simulink model "windEmulatorStep3"  (R2021a)
settings: Solver=ode4  StartTime=0.0  StopTime=inf  FixedStep=0.002  RelTol=1e-3
values from neighbouring files (symbols this model uses):
  ctrlModeSpeed = logical(false)    [initStep4.m]
  ctrlModeTorque = logical(true)    [initStep4.m]
  Dm_max = 40    [initStep4.m]
  EffMechMax = 0.93    [initStep4.m]
  EffMechMin = 0.79    [initStep4.m]
  FactorEff = psi2pa*cc2m3*(1/rev2rad)    (= 0.00109733470463)    [initStep4.m]
  genMaxTorque = 0.975*acs880RatedTorque    (= 78.48165)    [initStep4.m]
  Kdamping = -500    [OptimizationResultsLoad.m]
  Kpos = 0    [OptimizationResultsLoad.m]
  nPreDrop = 2900    [initStep4.m]
  nPreDropMin = 725    [initStep4.m]
  StatusWord = bitset(StatusWord,16)    [VFD_StatusWord.m]
  T = 4    [initStep4.m]
  wheelRadius = targetWaveBotVel/targetOmega    (= 0.00477464829276)    [initStep4.m]
undefined symbols (not defined in the file or in its folder): ACS880PILimLo, ACS880PILimUp, DiscIntNeverNeededParam, Gen_REF2_Max, Gen_SpeedScaling, minPressureRef, Motor_SpeedScaling, Motor_TorqueScaling, PressureControl, ratedTorque, rpm2rps, SpeedControl, speedScalingACS800, TorqueFieldbusScale, TorqueInputControl, TorqueRefMin
libraries: fl_lib x41, nesl_utility x24, slrealtimeethercatlib x21, sh_lib x16, cstblocks x4, simulink x3, pid_lib x3, sdl_lib x1, dspstat3 x1
(part 2 of 3)

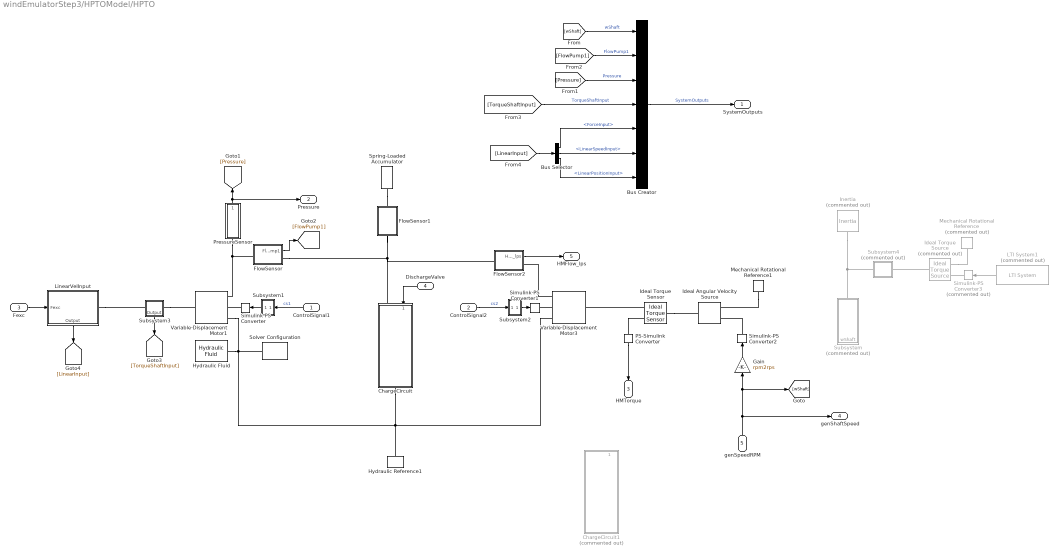
== system windEmulatorStep3/HPTOModel/HPTO ==
  ControlSignal1 : Inport
  ControlSignal2 : Inport  Port=2
  Fexc : Inport  Port=3
  DischargeValve : Inport  Port=4
  genSpeedRPM : Inport  Port=5
  Bus Creator : BusCreator  Inputs=7
  Bus Selector : BusSelector  OutputSignals=ForceInput,LinearSpeedInput,LinearPositionInput
  ChargeCircuit : Subsystem
      settings: PortSchema="{\"entries\":[{\"content\":{\"sides\":[{\"content\":{\"connectorIds\":[\"LConn1\",\"In1\"]},\"type\":\"ConnectorPlacement.EquallySpacedRectSide\",\"uuid\":\"82d1daf8-710b-4985-b266-be1c706fd037\"},{\"content\":{\"connectorIds\":[\"RConn1\"],\"side\":\"RIGHT\"},\"type\":\"ConnectorPlacement.EquallySpacedRectSide\",\"uuid\":\"cd9d67f9-1549-4eed-bef0-0a9dd1fc786d\"},{\"content\":{\"connectorIds\":[],\"side\":\"TOP\"},\"type\":\"ConnectorPlacement.EquallySpacedRectSide\",\"uuid\":\"e41a24c3-7fe9-4850-b669-e053dd15bed4\"},{\"content\":{\"connectorIds\":[],\"side\":\"BOTTOM\"},\"type\":\"ConnectorPlacement.EquallySpacedRectSide\",\"uuid\":\"127c729b-2c4a-40cb-ada2-aa7d7979a424\"}]},\"type\":\"ConnectorPlacement.EquallySpacedConnector\",\"uuid\":\"9c677d2b-4aa8-4aee-a320-3219a43d5bc8\"}],\"packageUris\":[\"http://schema.mathworks.com/mf0/Connector/R2020b\"],\"version\":\"1.0\"}"
  ChargeCircuit1 : Subsystem  Commented=on
      settings: PortSchema="{\"entries\":[{\"content\":{\"sides\":[{\"content\":{\"connectorIds\":[\"LConn1\",\"In1\"]},\"type\":\"ConnectorPlacement.EquallySpacedRectSide\",\"uuid\":\"82d1daf8-710b-4985-b266-be1c706fd037\"},{\"content\":{\"connectorIds\":[\"RConn1\"],\"side\":\"RIGHT\"},\"type\":\"ConnectorPlacement.EquallySpacedRectSide\",\"uuid\":\"cd9d67f9-1549-4eed-bef0-0a9dd1fc786d\"},{\"content\":{\"connectorIds\":[],\"side\":\"TOP\"},\"type\":\"ConnectorPlacement.EquallySpacedRectSide\",\"uuid\":\"e41a24c3-7fe9-4850-b669-e053dd15bed4\"},{\"content\":{\"connectorIds\":[\"RConn2\"],\"side\":\"BOTTOM\"},\"type\":\"ConnectorPlacement.EquallySpacedRectSide\",\"uuid\":\"127c729b-2c4a-40cb-ada2-aa7d7979a424\"}]},\"type\":\"ConnectorPlacement.EquallySpacedConnector\",\"uuid\":\"9c677d2b-4aa8-4aee-a320-3219a43d5bc8\"}],\"packageUris\":[\"http://schema.mathworks.com/mf0/Connector/R2020b\"],\"version\":\"1.0\"}"
  FlowSensor : Subsystem
  FlowSensor1 : Subsystem
  FlowSensor2 : Subsystem
  Gain : Gain  Gain=rpm2rps
  Hydraulic Fluid : sh_lib/Hydraulic Utilities/Hydraulic Fluid  DataSource=1  SelFluid=1  SysTemp=60  TrapAir=0.005  ViscDerFactor=1  range_error=1
  Hydraulic Reference1 : fl_lib/Hydraulic/Hydraulic Elements/Hydraulic Reference
  Ideal Angular Velocity Source : fl_lib/Mechanical/Mechanical Sources/Ideal Angular Velocity Source
  Ideal Torque Sensor : fl_lib/Mechanical/Mechanical Sensors/Ideal Torque Sensor
  Ideal Torque Source : fl_lib/Mechanical/Mechanical Sources/Ideal Torque Source  Commented=on
  Inertia : fl_lib/Mechanical/Rotational Elements/Inertia  Commented=on  inertia=1 kg*m^2  num_ports=foundation.enum.numPorts2.one  w_specify=off  w_priority=High  w=0 rpm  w_nominal_specify=off  w_nominal_unit=rad/s  w_nominal_value=1  t_specify=off  t_priority=None  t=0 N*m  t_nominal_specify=off  t_nominal_unit=N*m  t_nominal_value=1
  LTI System1 : cstblocks/LTI System  Commented=on  sys=tf(100*2*pi,[1 200*pi])  IC=[]
  LinearVelInput : Subsystem
      settings: PortSchema="{\"entries\":[{\"content\":{\"sides\":[{\"content\":{\"connectorIds\":[\"LConn1\"]},\"type\":\"ConnectorPlacement.EquallySpacedRectSide\",\"uuid\":\"4859a0f7-9f9b-474b-bb49-bd256c408622\"},{\"content\":{\"connectorIds\":[\"In1\"],\"side\":\"RIGHT\"},\"type\":\"ConnectorPlacement.EquallySpacedRectSide\",\"uuid\":\"5e25e59b-8f8b-4773-b6d9-951d4129523a\"},{\"content\":{\"connectorIds\":[],\"side\":\"TOP\"},\"type\":\"ConnectorPlacement.EquallySpacedRectSide\",\"uuid\":\"bae24e3d-e286-4bf4-a21b-122b1e5bc09f\"},{\"content\":{\"connectorIds\":[\"Out1\"],\"side\":\"BOTTOM\"},\"type\":\"ConnectorPlacement.EquallySpacedRectSide\",\"uuid\":\"0ce66b8b-3f3a-4f1a-9606-df56b31d9b3c\"}]},\"type\":\"ConnectorPlacement.EquallySpacedConnector\",\"uuid\":\"f87c39b6-c8d4-4afb-9096-6dab01ec5afa\"}],\"packageUris\":[\"http://schema.mathworks.com/mf0/Connector/R2020b\"],\"version\":\"1.0\"}"
  Mechanical Rotational Reference : fl_lib/Mechanical/Rotational Elements/Mechanical Rotational Reference  Commented=on
  Mechanical Rotational Reference1 : fl_lib/Mechanical/Rotational Elements/Mechanical Rotational Reference
  PS-Simulink Converter : nesl_utility/PS-Simulink Converter  PhysicalDomain=network_engine_domain  SubClassName=ps_output  LeftPortType=input  RightPortType=output  PseudoPeriodic=off  Frequencies=[]  Unit=inherit  AffineConversion=off
      settings: SourceProductBaseCode=PW,SS
  PressureSensor : Subsystem
  Simulink-PS Converter : nesl_utility/Simulink-PS Converter  PhysicalDomain=network_engine_domain  SubClassName=ps_input  LeftPortType=input  RightPortType=output  PseudoPeriodic=off  Frequencies=[]  NoiseDistribution=none  NoiseParameters=[]  Unit=1  AffineConversion=off  FilteringAndDerivatives=provide  SimscapeFilterOrder=1  InputFilterTimeConstant=0.001  UdotUserProvided=0
      settings: SourceProductBaseCode=PW,SS
  Simulink-PS Converter1 : nesl_utility/Simulink-PS Converter  PhysicalDomain=network_engine_domain  SubClassName=ps_input  LeftPortType=input  RightPortType=output  PseudoPeriodic=off  Frequencies=[]  NoiseDistribution=none  NoiseParameters=[]  Unit=1  AffineConversion=off  FilteringAndDerivatives=provide  SimscapeFilterOrder=1  InputFilterTimeConstant=0.001  UdotUserProvided=0
      settings: SourceProductBaseCode=PW,SS
  Simulink-PS Converter2 : nesl_utility/Simulink-PS Converter  PhysicalDomain=network_engine_domain  SubClassName=ps_input  LeftPortType=input  RightPortType=output  PseudoPeriodic=off  Frequencies=[]  NoiseDistribution=none  NoiseParameters=[]  Unit=1  AffineConversion=off  FilteringAndDerivatives=provide  SimscapeFilterOrder=1  InputFilterTimeConstant=0.001  UdotUserProvided=0
      settings: SourceProductBaseCode=PW,SS
  Simulink-PS Converter3 : nesl_utility/Simulink-PS Converter  Commented=on  PhysicalDomain=network_engine_domain  SubClassName=ps_input  LeftPortType=input  RightPortType=output  PseudoPeriodic=off  Frequencies=[]  NoiseDistribution=none  NoiseParameters=[]  Unit=1  AffineConversion=off  FilteringAndDerivatives=provide  SimscapeFilterOrder=1  InputFilterTimeConstant=0.001  UdotUserProvided=0
      settings: SourceProductBaseCode=PW,SS
  Solver Configuration : nesl_utility/Solver Configuration  PhysicalDomain=network_engine_domain  SubClassName=solver  LeftPortType=input  RightPortType=generic  Tones=[]  Harmonics=[]  SimulateNoise=off  Profile=off  UseLocalSampling=off  EnableSwitchedLinearOptims=on  FrequencyDomain=off  UseCCode=off  RelTol=0.001  AbsTol=1e-06  MinStep=1e-09  ToWorkspace=off  RevertToSquareIcSolve=off  NumHomotopyIterations=100  PhasorMode=off  PhasorModeNumHarmonics=1  DoDC=off  ResidualTolerance=1e-09  UseLocalSolver=on  LocalSolverChoice=NE_BACKWARD_EULER_ADVANCER  LocalSolverSampleTime=SampleTime  DoFixedCost=on  MaxNonlinIter=3  MaxModeIter=2  ComputeImpulses=off  ImpulseIterations=2  LinearAlgebra=auto  EquationFormulation=NE_TIME_EF  DelaysMemoryBudget=1024  AutomaticFiltering=on  FilteringTimeConstant=0.001  PartitionStorageMethod=AS_NEEDED  PartitionMemoryBudget=1024  PartitionMethod=ROBUST
      settings: SourceProductBaseCode=PW,SS
  Spring-Loaded Accumulator : sh_lib/Accumulators/Spring-Loaded Accumulator  capacity=AccVol m^3  pr_preload=Acc_PC psi  pr_max=Acc_MaxP psi  stiff_coeff=1e10 Pa/m^3  penetr_coeff=1e10 Pa*s/m^6  flow_rate_specify=off  flow_rate_priority=None  flow_rate=5e-3 m^3/s  flow_rate_nominal_specify=off  flow_rate_nominal_unit=m^3/s  flow_rate_nominal_value=1  fluid_volume_specify=on  fluid_volume_priority=None  fluid_volume=5e-6 m^3  fluid_volume_nominal_specify=off  fluid_volume_nominal_unit=m^3  fluid_volume_nominal_value=1  fluid_pressure_specify=off  fluid_pressure_priority=None  fluid_pressure=1.01325e5 Pa  fluid_pressure_nominal_specify=off  fluid_pressure_nominal_unit=Pa  fluid_pressure_nominal_value=1
      settings: SourceProductBaseCode=SH  InternalSimscapePortConfiguration="{\"Bottom\":[],\"Left\":[],\"Right\":[{\"id\":\"A\",\"label\":\"A\",\"type\":\"foundation.hydraulic.hydraulic\"}],\"Top\":[]}"
  Subsystem : Subsystem  Commented=on
  Subsystem1 : Subsystem
  Subsystem2 : Subsystem
  Subsystem3 : Subsystem
      settings: PortSchema="{\"entries\":[{\"content\":{\"sides\":[{\"content\":{\"connectorIds\":[\"LConn1\"]},\"type\":\"ConnectorPlacement.EquallySpacedRectSide\",\"uuid\":\"7d5827d5-19d2-449a-bfe5-3899d5f2f234\"},{\"content\":{\"connectorIds\":[\"RConn1\"],\"side\":\"RIGHT\"},\"type\":\"ConnectorPlacement.EquallySpacedRectSide\",\"uuid\":\"27ad7fb5-d235-43aa-a783-09c3ddbf3629\"},{\"content\":{\"connectorIds\":[],\"side\":\"TOP\"},\"type\":\"ConnectorPlacement.EquallySpacedRectSide\",\"uuid\":\"41db419c-7193-454e-a54e-cfb74ab94a84\"},{\"content\":{\"connectorIds\":[\"Out1\"],\"side\":\"BOTTOM\"},\"type\":\"ConnectorPlacement.EquallySpacedRectSide\",\"uuid\":\"63d69fbc-18e5-4f7b-99db-9fcc8740eddf\"}]},\"type\":\"ConnectorPlacement.EquallySpacedConnector\",\"uuid\":\"1d29a5fa-8394-444f-93a2-8698ce035363\"}],\"packageUris\":[\"http://schema.mathworks.com/mf0/Connector/R2020b\"],\"version\":\"1.0\"}"
  Subsystem4 : Subsystem  Commented=on
  Variable-Displacement Motor1 : sh_lib/Pumps and Motors/Variable-Displacement Motor  mdl_type=2  stroke_max=0.005 m  D_max=Dm_max cm^3/rev  cntrl_mem_tab=[-.0075, 0, .0075] m  displ_tab=[-Dm_max, 0, Dm_max] cm^3/rev  interp_method=1  extrap_method=1  loss_spec=1  w_nominal=nShaftSpeed rpm  pr_nominal=nPreDrop psi  visc_nominal=18 cSt  dens_nominal=900 kg/m^3  efficiency_vol=EffVolNom  no_load_torque=nTorqueNoLoad N*m  torque_pressure_coeff=(1/((200-50)*1e5))*Dm_max*FactorEff*((1-EffMechMax)*nPreDrop-(1-EffMechMin)*nPreDropMin) N*m/Pa  p_diff_eff_TLU=[100000, 1000000, 2000000] Pa  omega_eff_TLU=[25, 50, 100, 200, 300, 400] rad/s  displacement_eff_TLU=[-30, -19, 19, 30] cm^3/rev  vol_eff_TLU=repmat([.816, .908, .954, .977, .981, .984; .325, .663, .831, .916, .925, .946; .137, .568, .78, .892, .893, .91], 1, 1, 4)  mech_eff_TLU=repmat([.996, .996, .996, .996, .996, .996; .988, .989, .989, .989, .989, .99; .981, .981, .982, .982, .983, .984], 1, 1, 4)  p_diff_loss_TLU=[100000, 1000000, 2000000] Pa  omega_loss_TLU=[25, 50, 100, 200, 300, 400] rad/s  displacement_loss_TLU=[-30, -19, 19, 30] cm^3/rev  vol_loss_TLU=repmat([.0282, .0253, .0241, .0235, .0291, .0325; .2596, .1271, .1017, .0917, .1216, .1142; .7874, .1901, .141, .1211, .1797, .1978] * 1e-3, 1, 1, 4) m^3/s  mech_loss_TLU=repmat([.002, .002, .002, .002, .002, .002; .06, .055, .055, .055, .055, .05; .19, .19, .18, .18, .17, .16], 1, 1, 4) N*m  pressure_threshold=1e5 Pa  omega_threshold=10 rad/s  displacement_threshold=0.0001 cm^3/rev  octant_check=0  pressure_check=0  min_valid_pressure=0 Pa  vol_eff_min=1e-3  vol_eff_max=1  mech_eff_min=1e-3  mech_eff_max=1
      settings: SourceProductBaseCode=SH  InternalSimscapePortConfiguration="{\"Bottom\":[],\"Left\":[{\"id\":\"A\",\"label\":\"A\",\"type\":\"foundation.hydraulic.hydraulic\"},{\"id\":\"C\",\"label\":\"C\",\"type\":\"input\"},{\"id\":\"B\",\"label\":\"B\",\"type\":\"foundation.hydraulic.hydraulic\"}],\"Right\":[{\"id\":\"S\",\"label\":\"S\",\"type\":\"foundation.mechanical.rotational.rotational\"}],\"Top\":[]}"
  Variable-Displacement Motor3 : sh_lib/Pumps and Motors/Variable-Displacement Motor  mdl_type=2  stroke_max=0.005 m  D_max=Dm_max cm^3/rev  cntrl_mem_tab=[-.0075, 0, .0075] m  displ_tab=[-Dm_max, 0, Dm_max] cm^3/rev  interp_method=1  extrap_method=1  loss_spec=1  w_nominal=nShaftSpeed rpm  pr_nominal=nPreDrop psi  visc_nominal=18 cSt  dens_nominal=900 kg/m^3  efficiency_vol=EffVolNom  no_load_torque=nTorqueNoLoad N*m  torque_pressure_coeff=(1/((200-50)*1e5))*Dm_max*FactorEff*((1-EffMechMax)*nPreDrop-(1-EffMechMin)*nPreDropMin) N*m/Pa  p_diff_eff_TLU=[100000, 1000000, 2000000] Pa  omega_eff_TLU=[25, 50, 100, 200, 300, 400] rad/s  displacement_eff_TLU=[-30, -19, 19, 30] cm^3/rev  vol_eff_TLU=repmat([.816, .908, .954, .977, .981, .984; .325, .663, .831, .916, .925, .946; .137, .568, .78, .892, .893, .91], 1, 1, 4)  mech_eff_TLU=repmat([.996, .996, .996, .996, .996, .996; .988, .989, .989, .989, .989, .99; .981, .981, .982, .982, .983, .984], 1, 1, 4)  p_diff_loss_TLU=[100000, 1000000, 2000000] Pa  omega_loss_TLU=[25, 50, 100, 200, 300, 400] rad/s  displacement_loss_TLU=[-30, -19, 19, 30] cm^3/rev  vol_loss_TLU=repmat([.0282, .0253, .0241, .0235, .0291, .0325; .2596, .1271, .1017, .0917, .1216, .1142; .7874, .1901, .141, .1211, .1797, .1978] * 1e-3, 1, 1, 4) m^3/s  mech_loss_TLU=repmat([.002, .002, .002, .002, .002, .002; .06, .055, .055, .055, .055, .05; .19, .19, .18, .18, .17, .16], 1, 1, 4) N*m  pressure_threshold=1e5 Pa  omega_threshold=10 rad/s  displacement_threshold=0.00001 cm^3/rev  octant_check=0  pressure_check=0  min_valid_pressure=0 Pa  vol_eff_min=1e-3  vol_eff_max=1  mech_eff_min=1e-3  mech_eff_max=1
      settings: SourceProductBaseCode=SH  InternalSimscapePortConfiguration="{\"Bottom\":[],\"Left\":[{\"id\":\"A\",\"label\":\"A\",\"type\":\"foundation.hydraulic.hydraulic\"},{\"id\":\"C\",\"label\":\"C\",\"type\":\"input\"},{\"id\":\"B\",\"label\":\"B\",\"type\":\"foundation.hydraulic.hydraulic\"}],\"Right\":[{\"id\":\"S\",\"label\":\"S\",\"type\":\"foundation.mechanical.rotational.rotational\"}],\"Top\":[]}"
  SystemOutputs : Outport
  Pressure : Outport  Port=2
  HMTorque : Outport  Port=3
  genShaftSpeed : Outport  Port=4
  HMFlow_lps : Outport  Port=5
  wires:
  LTI System1/1 -> Simulink-PS Converter3/1
  [wShaft] -> Bus Creator/1  "wShaft"
  PressureSensor/1(Pressure) -> Pressure/1, [Pressure]
  Bus Creator/1 -> SystemOutputs/1  "SystemOutputs"
  ControlSignal1/1 -> Subsystem1/1(In1)  "cs1"
  Subsystem1/1(Out1) -> Simulink-PS Converter/1
  Subsystem2/1(Out1) -> Simulink-PS Converter1/1
  ControlSignal2/1 -> Subsystem2/1(1)  "cs2"
  FlowSensor/1(FlowPump1) -> [FlowPump1]
  [FlowPump1] -> Bus Creator/2  "FlowPump1"
  [Pressure] -> Bus Creator/3  "Pressure"
  Subsystem3/1(Output) -> [TorqueShaftInput]
  [TorqueShaftInput] -> Bus Creator/4  "TorqueShaftInput"
  LinearVelInput/1(Output) -> [LinearInput]
  [LinearInput] -> Bus Selector/1
  Bus Selector/2 -> Bus Creator/6  "<LinearSpeedInput>"
  Bus Selector/1 -> Bus Creator/5  "<ForceInput>"
  Bus Selector/3 -> Bus Creator/7  "<LinearPositionInput>"
  Fexc/1 -> LinearVelInput/1(Fexc)
  DischargeValve/1 -> ChargeCircuit/1(DischargeValve)
  Gain/1 -> Simulink-PS Converter2/1
  genSpeedRPM/1 -> [wShaft], Gain/1, genShaftSpeed/1
  PS-Simulink Converter/1 -> HMTorque/1
  FlowSensor2/1(HMFlow_lps) -> HMFlow_lps/1
  connections:
  Subsystem/LConn1 -- Subsystem4/RConn1 -- Inertia/LConn1
  FlowSensor1/LConn1 -- ChargeCircuit/LConn1 -- FlowSensor2/LConn1 -- FlowSensor/RConn1
  PressureSensor/LConn1 -- Variable-Displacement Motor1/LConn1 -- FlowSensor/LConn1
  Ideal Torque Source/RConn2 -- Mechanical Rotational Reference/LConn1
  Simulink-PS Converter3/RConn1 -- Ideal Torque Source/RConn1
  Variable-Displacement Motor3/LConn2 -- Simulink-PS Converter1/RConn1
  Simulink-PS Converter/RConn1 -- Variable-Displacement Motor1/LConn2
  Spring-Loaded Accumulator/RConn1 -- FlowSensor1/RConn1
  Variable-Displacement Motor3/LConn1 -- FlowSensor2/RConn1
  Subsystem3/RConn1 -- Variable-Displacement Motor1/RConn1
  LinearVelInput/LConn1 -- Subsystem3/LConn1
  Ideal Torque Source/LConn1 -- Subsystem4/LConn1
  Variable-Displacement Motor1/LConn3 -- Hydraulic Reference1/LConn1 -- ChargeCircuit/RConn1 -- Variable-Displacement Motor3/LConn3 -- Solver Configuration/RConn1 -- Hydraulic Fluid/RConn1
  Simulink-PS Converter2/RConn1 -- Ideal Angular Velocity Source/RConn1
  Mechanical Rotational Reference1/LConn1 -- Ideal Angular Velocity Source/RConn2
  Ideal Torque Sensor/LConn1 -- Ideal Angular Velocity Source/LConn1
  Ideal Torque Sensor/RConn1 -- Variable-Displacement Motor3/RConn1
  PS-Simulink Converter/LConn1 -- Ideal Torque Sensor/RConn2

== system windEmulatorStep3/HPTOModel/ControlAlgorithm/ForceToTorque ==
  ActualSignals : Inport
  Bus Selector : BusSelector  OutputSignals=LinearSpeedInput,LinearPositionInput
  Constant2 : Constant  Value=wheelRadius
  DesiredForce : Subsystem
  Gain : Gain  Gain=-1
  Product2 : Product
  TorqueD : Outport
  wires:
  ActualSignals/1 -> Bus Selector/1
  Product2/1 -> Gain/1
  Constant2/1 -> Product2/2
  Bus Selector/1 -> DesiredForce/1(<LinearSpeedInput>)  "<LinearSpeedInput>"
  Bus Selector/2 -> DesiredForce/2(<LinearPositionInput>)  "<LinearPositionInput>"
  DesiredForce/1(ForceD) -> Product2/1
  Gain/1 -> TorqueD/1

== system windEmulatorStep3/HPTOModel/ControlAlgorithm/PressureAbovePmin ==
  ActualSignals : Inport
  RefValues : Inport  Port=2
  SpeedControllerReset : Inport  Port=3
  Bus Selector : BusSelector  OutputSignals=TorqueShaftInput,Pressure,wShaft
  Bus Selector1 : BusSelector  OutputSignals=TorqueInputRef,PressureRef,SheftSpeedRef
  PressureControl1 : Subsystem
  SpeedControl1 : Subsystem
  Terminator1 : Terminator
  TorqueControl1 : Subsystem
  ControlSignal1 : Outport
  ControlSignal2 : Outport  Port=2
  ControlTorqueLoad : Outport  Port=3
  wires:
  ActualSignals/1 -> Bus Selector/1
  TorqueControl1/1(ControlSignal1) -> ControlSignal1/1
  Bus Selector/3 -> SpeedControl1/1(ShaftSpeedMotor)  "<wShaft>"
  RefValues/1 -> Bus Selector1/1
  Bus Selector1/1 -> TorqueControl1/1(TorqueRef)  "<TorqueInputRef>"
  Bus Selector1/3 -> SpeedControl1/2(ShaftSpeedRef)  "<SheftSpeedRef>"
  PressureControl1/1(ControlSignal2) -> ControlSignal2/1
  Bus Selector/2 -> PressureControl1/1(ActualPressure)  "<Pressure>"
  Bus Selector/1 -> Terminator1/1  "<TorqueShaftInput>"
  Bus Selector1/2 -> PressureControl1/2(PressureRef)  "<PressureRef>"
  SpeedControl1/1(ContolTorque) -> ControlTorqueLoad/1
  SpeedControllerReset/1 -> SpeedControl1/3(SpeedControllerReset)

== system windEmulatorStep3/HPTOModel/ControlAlgorithm/PressureBelowPmin ==
  ActualSignals : Inport
  RefValues : Inport  Port=2
  SpeedControllerReset : Inport  Port=3
  Bus Selector : BusSelector  OutputSignals=TorqueShaftInput,Pressure,wShaft
  Bus Selector1 : BusSelector  OutputSignals=TorqueInputRef,PressureRef,SheftSpeedRef
  PressureControl1 : Subsystem
  SpeedControl1 : Subsystem
  TorqueControl1 : Subsystem
  ControlSignal1 : Outport
  ControlSignal2 : Outport  Port=2
  ControlTorqueLoad : Outport  Port=3
  wires:
  ActualSignals/1 -> Bus Selector/1
  Bus Selector/1 -> TorqueControl1/1(ActualTorqueInput)  "<TorqueShaftInput>"
  TorqueControl1/1(ControlSignal1) -> ControlSignal1/1
  PressureControl1/1(ControlSignal2) -> ControlSignal2/1
  Bus Selector/2 -> TorqueControl1/3(Pressure), PressureControl1/1(ActualPressure)  "<Pressure>"
  Bus Selector/3 -> SpeedControl1/1(ShaftSpeedMotor)  "<wShaft>"
  SpeedControl1/1(ContolTorque) -> ControlTorqueLoad/1
  RefValues/1 -> Bus Selector1/1
  Bus Selector1/1 -> TorqueControl1/2(TorqueRef)  "<TorqueInputRef>"
  Bus Selector1/2 -> PressureControl1/2(PressureRef)  "<PressureRef>"
  Bus Selector1/3 -> SpeedControl1/2(ShaftSpeedRef)  "<SheftSpeedRef>"
  SpeedControllerReset/1 -> SpeedControl1/3(SpeedControllerReset)

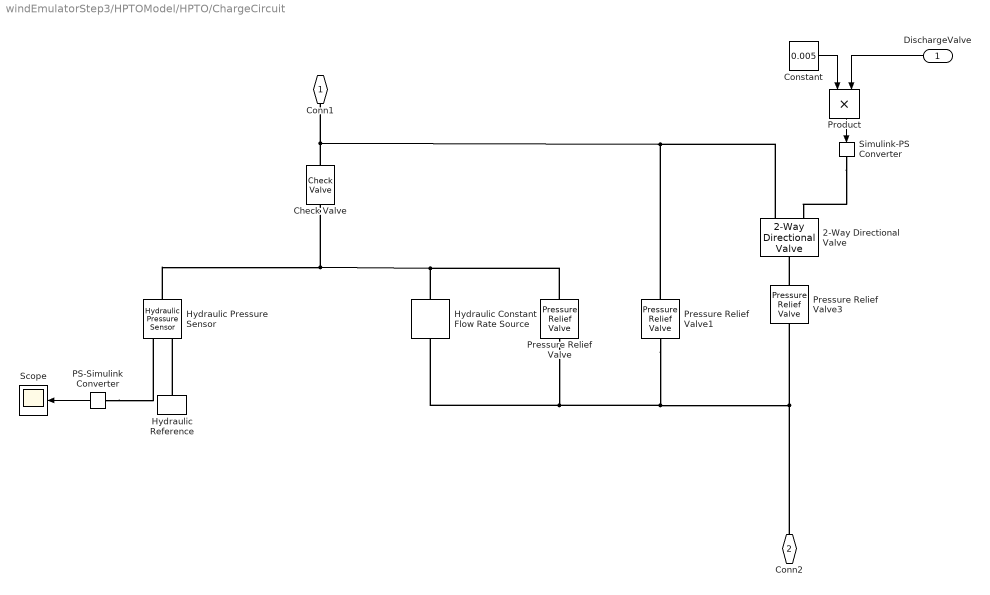
== system windEmulatorStep3/HPTOModel/HPTO/ChargeCircuit ==
  DischargeValve : Inport
  2-Way Directional Valve : sh_lib/Valves/Directional Valves/2-Way Directional Valve  mdl_type=1  area_max=0.5e-4 m^2  opening_max=0.005 m  opening_tab=[-.002, 0, .002, .005, .015] m  area_tab=[1e-09, 2.0352e-07, 4.0736e-05, .00011438, .00034356] m^2  pressure_tab=[-10000000, -5000000, -2000000, 2000000, 5000000, 10000000] Pa  flow_rate_tab=[-1e-07, -7.0711e-08, -4.4721e-08, 4.4721e-08, 7.0711e-08, 1e-07; -2.0352e-05, -1.4391e-05, -9.1017e-06, 9.1017e-06, 1.4391e-05, 2.0352e-05; -.0040736, -.0028805, -.0018218, .0018218, .0028805, .0040736; -.011438, -.0080879, -.0051152, .0051152, .0080879, .011438; -.034356, -.024293, -.015364, .015364, .024293, .034356] m^3/s  interp_method=1  extrap_method=1  C_d=0.7  x_0=0 m  A_leak=1e-12 m^2  lam_spec=1  B_lam=0.999  Re_cr=12
      settings: SourceProductBaseCode=SH  InternalSimscapePortConfiguration="{\"Bottom\":[],\"Left\":[{\"id\":\"S\",\"label\":\"S\",\"type\":\"input\"},{\"id\":\"A\",\"label\":\"A\",\"type\":\"foundation.hydraulic.hydraulic\"}],\"Right\":[{\"id\":\"B\",\"label\":\"B\",\"type\":\"foundation.hydraulic.hydraulic\"}],\"Top\":[]}"
  Check Valve : sh_lib/Valves/Directional Valves/Check Valve  area_max=1e-4 m^2  pres_crack=0.3e5 Pa  pres_max=1.2e5 Pa  C_d=0.7  A_leak=1e-12 m^2  lam_spec=1  B_lam=0.999  Re_cr=12  dynamic=0  tau=0.1 s  area_init=1e-12 m^2
      settings: SourceProductBaseCode=SH  InternalSimscapePortConfiguration="{\"Bottom\":[],\"Left\":[{\"id\":\"A\",\"label\":\"A\",\"type\":\"foundation.hydraulic.hydraulic\"}],\"Right\":[{\"id\":\"B\",\"label\":\"B\",\"type\":\"foundation.hydraulic.hydraulic\"}],\"Top\":[]}"
  Constant : Constant  Value=0.005
  Hydraulic Constant Flow Rate Source : fl_lib/Hydraulic/Hydraulic Sources/Hydraulic Constant Flow Rate Source  commanded_flow_rate=5 lpm
      settings: SourceProductBaseCode=SS  InternalSimscapePortConfiguration="{\"Bottom\":[],\"Left\":[{\"id\":\"P\",\"label\":\"P\",\"type\":\"foundation.hydraulic.hydraulic\"}],\"Right\":[{\"id\":\"T\",\"label\":\"T\",\"type\":\"foundation.hydraulic.hydraulic\"}],\"Top\":[]}"
  Hydraulic Pressure Sensor : fl_lib/Hydraulic/Hydraulic Sensors/Hydraulic Pressure Sensor
  Hydraulic Reference : fl_lib/Hydraulic/Hydraulic Elements/Hydraulic Reference
  PS-Simulink Converter : nesl_utility/PS-Simulink Converter  PhysicalDomain=network_engine_domain  SubClassName=ps_output  LeftPortType=input  RightPortType=output  PseudoPeriodic=off  Frequencies=[]  Unit=inherit  AffineConversion=off
      settings: SourceProductBaseCode=PW,SS
  Pressure Relief Valve : sh_lib/Valves/Pressure Control Valves/Pressure Relief Valve  valve_area_spec=1  p_diff_TLU=[30.15e5 : 15e3 : 31.35e5] Pa  area_TLU=[1 : 1 : 9] .* 1e-5 m^2  area_max=1e-4 m^2  pres_set=10 psi  reg_range=5 psi  C_d=0.7  A_leak=1e-12 m^2  lam_spec=1  B_lam=0.999  Re_cr=12  dynamic=0  tau=0.1 s  area_init=1e-12 m^2
      settings: SourceProductBaseCode=SH  InternalSimscapePortConfiguration="{\"Bottom\":[],\"Left\":[{\"id\":\"A\",\"label\":\"A\",\"type\":\"foundation.hydraulic.hydraulic\"}],\"Right\":[{\"id\":\"B\",\"label\":\"B\",\"type\":\"foundation.hydraulic.hydraulic\"}],\"Top\":[]}"
  Pressure Relief Valve1 : sh_lib/Valves/Pressure Control Valves/Pressure Relief Valve  valve_area_spec=1  p_diff_TLU=[30.15e5 : 15e3 : 31.35e5] Pa  area_TLU=[1 : 1 : 9] .* 1e-5 m^2  area_max=1e-4 m^2  pres_set=PressureValveMax psi  reg_range=ValvePreRange psi  C_d=0.7  A_leak=1e-12 m^2  lam_spec=1  B_lam=0.999  Re_cr=12  dynamic=0  tau=0.1 s  area_init=1e-12 m^2
      settings: SourceProductBaseCode=SH  InternalSimscapePortConfiguration="{\"Bottom\":[],\"Left\":[{\"id\":\"A\",\"label\":\"A\",\"type\":\"foundation.hydraulic.hydraulic\"}],\"Right\":[{\"id\":\"B\",\"label\":\"B\",\"type\":\"foundation.hydraulic.hydraulic\"}],\"Top\":[]}"
  Pressure Relief Valve3 : sh_lib/Valves/Pressure Control Valves/Pressure Relief Valve  valve_area_spec=1  p_diff_TLU=[30.15e5 : 15e3 : 31.35e5] Pa  area_TLU=[1 : 1 : 9] .* 1e-5 m^2  area_max=1e-4 m^2  pres_set=50 psi  reg_range=5 psi  C_d=0.7  A_leak=1e-12 m^2  lam_spec=1  B_lam=0.999  Re_cr=12  dynamic=0  tau=0.1 s  area_init=1e-12 m^2
      settings: SourceProductBaseCode=SH  InternalSimscapePortConfiguration="{\"Bottom\":[],\"Left\":[{\"id\":\"A\",\"label\":\"A\",\"type\":\"foundation.hydraulic.hydraulic\"}],\"Right\":[{\"id\":\"B\",\"label\":\"B\",\"type\":\"foundation.hydraulic.hydraulic\"}],\"Top\":[]}"
  Product : Product
  Scope : Scope
  Simulink-PS Converter : nesl_utility/Simulink-PS Converter  PhysicalDomain=network_engine_domain  SubClassName=ps_input  LeftPortType=input  RightPortType=output  PseudoPeriodic=off  Frequencies=[]  NoiseDistribution=none  NoiseParameters=[]  Unit=1  AffineConversion=off  FilteringAndDerivatives=provide  SimscapeFilterOrder=1  InputFilterTimeConstant=0.001  UdotUserProvided=0
      settings: SourceProductBaseCode=PW,SS
  Conn1 : PMIOPort  Side=Left
  Conn2 : PMIOPort  Port=2  Side=Right
  wires:
  PS-Simulink Converter/1 -> Scope/1
  Product/1 -> Simulink-PS Converter/1
  Constant/1 -> Product/1
  DischargeValve/1 -> Product/2
  connections:
  Hydraulic Pressure Sensor/LConn1 -- Pressure Relief Valve/LConn1 -- Hydraulic Constant Flow Rate Source/LConn1 -- Check Valve/LConn1
  Hydraulic Constant Flow Rate Source/RConn1 -- Pressure Relief Valve1/RConn1 -- Conn2/RConn1 -- Pressure Relief Valve3/RConn1 -- Pressure Relief Valve/RConn1
  Check Valve/RConn1 -- 2-Way Directional Valve/LConn2 -- Pressure Relief Valve1/LConn1 -- Conn1/RConn1
  Hydraulic Reference/LConn1 -- Hydraulic Pressure Sensor/RConn1
  PS-Simulink Converter/LConn1 -- Hydraulic Pressure Sensor/RConn2
  Simulink-PS Converter/RConn1 -- 2-Way Directional Valve/LConn1
  Pressure Relief Valve3/LConn1 -- 2-Way Directional Valve/RConn1

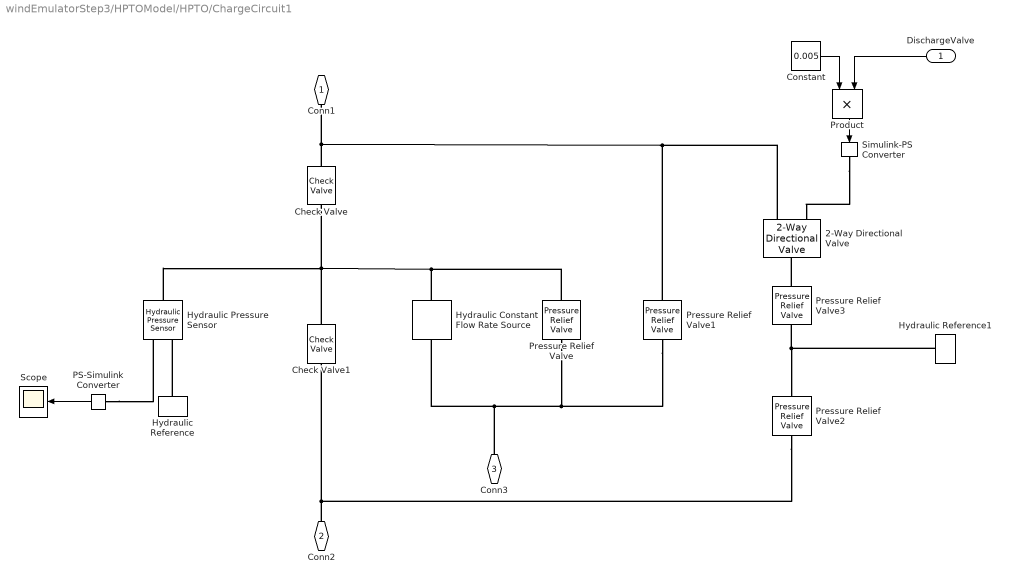
== system windEmulatorStep3/HPTOModel/HPTO/ChargeCircuit1 ==
  DischargeValve : Inport
  2-Way Directional Valve : sh_lib/Valves/Directional Valves/2-Way Directional Valve  mdl_type=1  area_max=0.5e-4 m^2  opening_max=0.005 m  opening_tab=[-.002, 0, .002, .005, .015] m  area_tab=[1e-09, 2.0352e-07, 4.0736e-05, .00011438, .00034356] m^2  pressure_tab=[-10000000, -5000000, -2000000, 2000000, 5000000, 10000000] Pa  flow_rate_tab=[-1e-07, -7.0711e-08, -4.4721e-08, 4.4721e-08, 7.0711e-08, 1e-07; -2.0352e-05, -1.4391e-05, -9.1017e-06, 9.1017e-06, 1.4391e-05, 2.0352e-05; -.0040736, -.0028805, -.0018218, .0018218, .0028805, .0040736; -.011438, -.0080879, -.0051152, .0051152, .0080879, .011438; -.034356, -.024293, -.015364, .015364, .024293, .034356] m^3/s  interp_method=1  extrap_method=1  C_d=0.7  x_0=0 m  A_leak=1e-12 m^2  lam_spec=1  B_lam=0.999  Re_cr=12
      settings: SourceProductBaseCode=SH  InternalSimscapePortConfiguration="{\"Bottom\":[],\"Left\":[{\"id\":\"S\",\"label\":\"S\",\"type\":\"input\"},{\"id\":\"A\",\"label\":\"A\",\"type\":\"foundation.hydraulic.hydraulic\"}],\"Right\":[{\"id\":\"B\",\"label\":\"B\",\"type\":\"foundation.hydraulic.hydraulic\"}],\"Top\":[]}"
  Check Valve : sh_lib/Valves/Directional Valves/Check Valve  area_max=1e-4 m^2  pres_crack=0.3e5 Pa  pres_max=1.2e5 Pa  C_d=0.7  A_leak=1e-12 m^2  lam_spec=1  B_lam=0.999  Re_cr=12  dynamic=0  tau=0.1 s  area_init=1e-12 m^2
      settings: SourceProductBaseCode=SH  InternalSimscapePortConfiguration="{\"Bottom\":[],\"Left\":[{\"id\":\"A\",\"label\":\"A\",\"type\":\"foundation.hydraulic.hydraulic\"}],\"Right\":[{\"id\":\"B\",\"label\":\"B\",\"type\":\"foundation.hydraulic.hydraulic\"}],\"Top\":[]}"
  Check Valve1 : sh_lib/Valves/Directional Valves/Check Valve  area_max=1e-4 m^2  pres_crack=0.3e5 Pa  pres_max=1.2e5 Pa  C_d=0.7  A_leak=1e-12 m^2  lam_spec=1  B_lam=0.999  Re_cr=12  dynamic=0  tau=0.1 s  area_init=1e-12 m^2
      settings: SourceProductBaseCode=SH  InternalSimscapePortConfiguration="{\"Bottom\":[],\"Left\":[{\"id\":\"A\",\"label\":\"A\",\"type\":\"foundation.hydraulic.hydraulic\"}],\"Right\":[{\"id\":\"B\",\"label\":\"B\",\"type\":\"foundation.hydraulic.hydraulic\"}],\"Top\":[]}"
  Constant : Constant  Value=0.005
  Hydraulic Constant Flow Rate Source : fl_lib/Hydraulic/Hydraulic Sources/Hydraulic Constant Flow Rate Source  commanded_flow_rate=35 lpm
      settings: SourceProductBaseCode=SS  InternalSimscapePortConfiguration="{\"Bottom\":[],\"Left\":[{\"id\":\"P\",\"label\":\"P\",\"type\":\"foundation.hydraulic.hydraulic\"}],\"Right\":[{\"id\":\"T\",\"label\":\"T\",\"type\":\"foundation.hydraulic.hydraulic\"}],\"Top\":[]}"
  Hydraulic Pressure Sensor : fl_lib/Hydraulic/Hydraulic Sensors/Hydraulic Pressure Sensor
  Hydraulic Reference : fl_lib/Hydraulic/Hydraulic Elements/Hydraulic Reference
  Hydraulic Reference1 : fl_lib/Hydraulic/Hydraulic Elements/Hydraulic Reference
  PS-Simulink Converter : nesl_utility/PS-Simulink Converter  PhysicalDomain=network_engine_domain  SubClassName=ps_output  LeftPortType=input  RightPortType=output  PseudoPeriodic=off  Frequencies=[]  Unit=inherit  AffineConversion=off
      settings: SourceProductBaseCode=PW,SS
  Pressure Relief Valve : sh_lib/Valves/Pressure Control Valves/Pressure Relief Valve  valve_area_spec=1  p_diff_TLU=[30.15e5 : 15e3 : 31.35e5] Pa  area_TLU=[1 : 1 : 9] .* 1e-5 m^2  area_max=1e-4 m^2  pres_set=50 psi  reg_range=5 psi  C_d=0.7  A_leak=1e-12 m^2  lam_spec=1  B_lam=0.999  Re_cr=12  dynamic=0  tau=0.1 s  area_init=1e-12 m^2
      settings: SourceProductBaseCode=SH  InternalSimscapePortConfiguration="{\"Bottom\":[],\"Left\":[{\"id\":\"A\",\"label\":\"A\",\"type\":\"foundation.hydraulic.hydraulic\"}],\"Right\":[{\"id\":\"B\",\"label\":\"B\",\"type\":\"foundation.hydraulic.hydraulic\"}],\"Top\":[]}"
  Pressure Relief Valve1 : sh_lib/Valves/Pressure Control Valves/Pressure Relief Valve  valve_area_spec=1  p_diff_TLU=[30.15e5 : 15e3 : 31.35e5] Pa  area_TLU=[1 : 1 : 9] .* 1e-5 m^2  area_max=1e-4 m^2  pres_set=PressureValveMax psi  reg_range=ValvePreRange psi  C_d=0.7  A_leak=1e-12 m^2  lam_spec=1  B_lam=0.999  Re_cr=12  dynamic=0  tau=0.1 s  area_init=1e-12 m^2
      settings: SourceProductBaseCode=SH  InternalSimscapePortConfiguration="{\"Bottom\":[],\"Left\":[{\"id\":\"A\",\"label\":\"A\",\"type\":\"foundation.hydraulic.hydraulic\"}],\"Right\":[{\"id\":\"B\",\"label\":\"B\",\"type\":\"foundation.hydraulic.hydraulic\"}],\"Top\":[]}"
  Pressure Relief Valve2 : sh_lib/Valves/Pressure Control Valves/Pressure Relief Valve  valve_area_spec=1  p_diff_TLU=[30.15e5 : 15e3 : 31.35e5] Pa  area_TLU=[1 : 1 : 9] .* 1e-5 m^2  area_max=1e-4 m^2  pres_set=PressureValveMax psi  reg_range=ValvePreRange psi  C_d=0.7  A_leak=1e-12 m^2  lam_spec=1  B_lam=0.999  Re_cr=12  dynamic=0  tau=0.1 s  area_init=1e-12 m^2
      settings: SourceProductBaseCode=SH  InternalSimscapePortConfiguration="{\"Bottom\":[],\"Left\":[{\"id\":\"A\",\"label\":\"A\",\"type\":\"foundation.hydraulic.hydraulic\"}],\"Right\":[{\"id\":\"B\",\"label\":\"B\",\"type\":\"foundation.hydraulic.hydraulic\"}],\"Top\":[]}"
  Pressure Relief Valve3 : sh_lib/Valves/Pressure Control Valves/Pressure Relief Valve  valve_area_spec=1  p_diff_TLU=[30.15e5 : 15e3 : 31.35e5] Pa  area_TLU=[1 : 1 : 9] .* 1e-5 m^2  area_max=1e-4 m^2  pres_set=50 psi  reg_range=5 psi  C_d=0.7  A_leak=1e-12 m^2  lam_spec=1  B_lam=0.999  Re_cr=12  dynamic=0  tau=0.1 s  area_init=1e-12 m^2
      settings: SourceProductBaseCode=SH  InternalSimscapePortConfiguration="{\"Bottom\":[],\"Left\":[{\"id\":\"A\",\"label\":\"A\",\"type\":\"foundation.hydraulic.hydraulic\"}],\"Right\":[{\"id\":\"B\",\"label\":\"B\",\"type\":\"foundation.hydraulic.hydraulic\"}],\"Top\":[]}"
  Product : Product
  Scope : Scope
  Simulink-PS Converter : nesl_utility/Simulink-PS Converter  PhysicalDomain=network_engine_domain  SubClassName=ps_input  LeftPortType=input  RightPortType=output  PseudoPeriodic=off  Frequencies=[]  NoiseDistribution=none  NoiseParameters=[]  Unit=1  AffineConversion=off  FilteringAndDerivatives=provide  SimscapeFilterOrder=1  InputFilterTimeConstant=0.001  UdotUserProvided=0
      settings: SourceProductBaseCode=PW,SS
  Conn1 : PMIOPort  Side=Left
  Conn2 : PMIOPort  Port=2  Side=Right
  Conn3 : PMIOPort  Port=3  Side=Right
  wires:
  PS-Simulink Converter/1 -> Scope/1
  Product/1 -> Simulink-PS Converter/1
  Constant/1 -> Product/1
  DischargeValve/1 -> Product/2
  connections:
  Check Valve1/LConn1 -- Hydraulic Pressure Sensor/LConn1 -- Pressure Relief Valve/LConn1 -- Hydraulic Constant Flow Rate Source/LConn1 -- Check Valve/LConn1
  Conn2/RConn1 -- Pressure Relief Valve2/LConn1 -- Check Valve1/RConn1
  Check Valve/RConn1 -- 2-Way Directional Valve/LConn2 -- Pressure Relief Valve1/LConn1 -- Conn1/RConn1
  Conn3/RConn1 -- Pressure Relief Valve1/RConn1 -- Pressure Relief Valve/RConn1 -- Hydraulic Constant Flow Rate Source/RConn1
  Hydraulic Reference/LConn1 -- Hydraulic Pressure Sensor/RConn1
  PS-Simulink Converter/LConn1 -- Hydraulic Pressure Sensor/RConn2
  Hydraulic Reference1/LConn1 -- Pressure Relief Valve3/RConn1 -- Pressure Relief Valve2/RConn1
  Simulink-PS Converter/RConn1 -- 2-Way Directional Valve/LConn1
  Pressure Relief Valve3/LConn1 -- 2-Way Directional Valve/RConn1

== system windEmulatorStep3/HPTOModel/HPTO/FlowSensor ==
  Hydraulic Flow Rate Sensor : fl_lib/Hydraulic/Hydraulic Sensors/Hydraulic Flow Rate Sensor
  PS Terminator : fl_lib/Physical Signals/Sinks/PS Terminator
  PS-Simulink Converter : nesl_utility/PS-Simulink Converter  PhysicalDomain=network_engine_domain  SubClassName=ps_output  LeftPortType=input  RightPortType=output  PseudoPeriodic=off  Frequencies=[]  Unit=inherit  AffineConversion=off
      settings: SourceProductBaseCode=PW,SS
  Scope : Scope
  m3toL : Gain  Gain=1000*60
  Qin : PMIOPort  Side=Left
  Qout : PMIOPort  Port=2  Side=Right
  FlowPump1 : Outport
  wires:
  PS-Simulink Converter/1 -> m3toL/1, Scope/1
  m3toL/1 -> FlowPump1/1  "FlowPump1"
  connections:
  PS-Simulink Converter/LConn1 -- Hydraulic Flow Rate Sensor/RConn1
  Hydraulic Flow Rate Sensor/RConn2 -- Qout/RConn1
  PS Terminator/LConn1 -- Hydraulic Flow Rate Sensor/RConn3
  Hydraulic Flow Rate Sensor/LConn1 -- Qin/RConn1

== system windEmulatorStep3/HPTOModel/HPTO/FlowSensor1 ==
  Gain : Gain  Gain=1000*60
  Hydraulic Flow Rate Sensor : fl_lib/Hydraulic/Hydraulic Sensors/Hydraulic Flow Rate Sensor
  PS Terminator : fl_lib/Physical Signals/Sinks/PS Terminator
  PS-Simulink Converter : nesl_utility/PS-Simulink Converter  PhysicalDomain=network_engine_domain  SubClassName=ps_output  LeftPortType=input  RightPortType=output  PseudoPeriodic=off  Frequencies=[]  Unit=inherit  AffineConversion=off
      settings: SourceProductBaseCode=PW,SS
  Scope : Scope
  Qin : PMIOPort  Side=Left
  Qout : PMIOPort  Port=2  Side=Right
  wires:
  PS-Simulink Converter/1 -> Gain/1
  Gain/1 -> Scope/1  "FlowAccumulator"
  connections:
  PS-Simulink Converter/LConn1 -- Hydraulic Flow Rate Sensor/RConn1
  Hydraulic Flow Rate Sensor/RConn2 -- Qout/RConn1
  PS Terminator/LConn1 -- Hydraulic Flow Rate Sensor/RConn3
  Hydraulic Flow Rate Sensor/LConn1 -- Qin/RConn1

== system windEmulatorStep3/HPTOModel/HPTO/FlowSensor2 ==
  Gain : Gain  Gain=1000*60
  Hydraulic Flow Rate Sensor : fl_lib/Hydraulic/Hydraulic Sensors/Hydraulic Flow Rate Sensor
  PS Terminator : fl_lib/Physical Signals/Sinks/PS Terminator
  PS-Simulink Converter : nesl_utility/PS-Simulink Converter  PhysicalDomain=network_engine_domain  SubClassName=ps_output  LeftPortType=input  RightPortType=output  PseudoPeriodic=off  Frequencies=[]  Unit=inherit  AffineConversion=off
      settings: SourceProductBaseCode=PW,SS
  Scope : Scope
  Qin : PMIOPort  Side=Left
  Qout : PMIOPort  Port=2  Side=Right
  HMFlow_lps : Outport
  wires:
  PS-Simulink Converter/1 -> Gain/1
  Gain/1 -> HMFlow_lps/1, Scope/1  "FlowMotor1"
  connections:
  PS-Simulink Converter/LConn1 -- Hydraulic Flow Rate Sensor/RConn1
  Hydraulic Flow Rate Sensor/RConn2 -- Qout/RConn1
  PS Terminator/LConn1 -- Hydraulic Flow Rate Sensor/RConn3
  Hydraulic Flow Rate Sensor/LConn1 -- Qin/RConn1

== system windEmulatorStep3/HPTOModel/HPTO/LinearVelInput ==
  Fexc : Inport
  Gear Box : fl_lib/Mechanical/Mechanisms/Gear Box  Commented=on  ratio=GearRatio  t_in_specify=off  t_in_priority=None  t_in=0 N*m  t_in_nominal_specify=off  t_in_nominal_unit=N*m  t_in_nominal_value=1  t_out_specify=off  t_out_priority=None  t_out=0 N*m  t_out_nominal_specify=off  t_out_nominal_unit=N*m  t_out_nominal_value=1
  Ideal Force Sensor1 : fl_lib/Mechanical/Mechanical Sensors/Ideal Force Sensor
  PS-Simulink Converter : nesl_utility/PS-Simulink Converter  PhysicalDomain=network_engine_domain  SubClassName=ps_output  LeftPortType=input  RightPortType=output  PseudoPeriodic=off  Frequencies=[]  Unit=inherit  AffineConversion=off
      settings: SourceProductBaseCode=PW,SS
  Rack & Pinion : sdl_lib/Gears/Rotational- Translational/Rack & Pinion  Commented=on  param=sdl.enum.rackPinionParameters.radius  radius=P_radius m  n_teeth=20  x_tooth=5 mm  rack_direction_sign=sdl.enum.pinionDirection.positive  friction_model=sdl.enum.gear_friction.none  mu_visc_P=0 N*m/(rad/s)  mu_visc_R=0 N/(m/s)  efficiency=0.8  temperature_TLU=[280, 300, 320] K  efficiency_TLU=[.95, .9, .85]  pwr_thr=0.001 W  thermal_mass=50 J/K  temperature_specify=off  temperature_priority=High  temperature=300 K  temperature_nominal_specify=off  temperature_nominal_unit=K  temperature_nominal_value=1
      settings: SourceProductBaseCode=LD  InternalSimscapePortConfiguration="{\"Bottom\":[],\"Left\":[{\"id\":\"P\",\"label\":\"P\",\"type\":\"foundation.mechanical.rotational.rotational\"}],\"Right\":[{\"id\":\"R\",\"label\":\"R\",\"type\":\"foundation.mechanical.translational.translational\"}],\"Top\":[]}"
  Subsystem : Subsystem
      settings: PortSchema="{\"entries\":[{\"content\":{\"sides\":[{\"content\":{\"connectorIds\":[\"LConn1\"]},\"type\":\"ConnectorPlacement.EquallySpacedRectSide\",\"uuid\":\"215b7bca-b171-42a0-8110-3ac7d91926b2\"},{\"content\":{\"connectorIds\":[\"RConn1\"],\"side\":\"RIGHT\"},\"type\":\"ConnectorPlacement.EquallySpacedRectSide\",\"uuid\":\"231e152d-bce3-44d9-a550-7c1231ef5d98\"},{\"content\":{\"connectorIds\":[],\"side\":\"TOP\"},\"type\":\"ConnectorPlacement.EquallySpacedRectSide\",\"uuid\":\"bc851d42-4603-42fa-9c49-ea05891b2ab9\"},{\"content\":{\"connectorIds\":[\"Out1\"],\"side\":\"BOTTOM\"},\"type\":\"ConnectorPlacement.EquallySpacedRectSide\",\"uuid\":\"67c0fa27-8a6c-4f46-81b7-2dea8cbe6936\"}]},\"type\":\"ConnectorPlacement.EquallySpacedConnector\",\"uuid\":\"7442d2b0-500a-4e34-82e4-4fa764ec5830\"}],\"packageUris\":[\"http://schema.mathworks.com/mf0/Connector/R2020b\"],\"version\":\"1.0\"}"
  WavebotModel : Subsystem
  Wheel and Axle : fl_lib/Mechanical/Mechanisms/Wheel and Axle  R=wheelRadius m  or=1  t_specify=off  t_priority=None  t=0 N*m  t_nominal_specify=off  t_nominal_unit=N*m  t_nominal_value=1  f_specify=off  f_priority=None  f=0 N  f_nominal_specify=off  f_nominal_unit=N  f_nominal_value=1
  Shaft : PMIOPort  Side=Left
  Output : Outport
  wires:
  Subsystem/1(LinearInput) -> Output/1
  PS-Simulink Converter/1 -> WavebotModel/1(PTOForce)
  Fexc/1 -> WavebotModel/2(Fexc)
  connections:
  Rack & Pinion/LConn1 -- Gear Box/LConn1
  PS-Simulink Converter/LConn1 -- Ideal Force Sensor1/RConn2
  WavebotModel/RConn1 -- Ideal Force Sensor1/RConn1
  Subsystem/LConn1 -- Ideal Force Sensor1/LConn1
  Wheel and Axle/RConn1 -- Subsystem/RConn1
  Wheel and Axle/LConn1 -- Shaft/RConn1

== system windEmulatorStep3/HPTOModel/HPTO/PressureSensor ==
  Gain : Gain  Gain=1/6894.75
  Hydraulic Pressure Sensor : fl_lib/Hydraulic/Hydraulic Sensors/Hydraulic Pressure Sensor
  Hydraulic Reference2 : fl_lib/Hydraulic/Hydraulic Elements/Hydraulic Reference
  PS-Simulink Converter : nesl_utility/PS-Simulink Converter  PhysicalDomain=network_engine_domain  SubClassName=ps_output  LeftPortType=input  RightPortType=output  PseudoPeriodic=off  Frequencies=[]  Unit=inherit  AffineConversion=off
      settings: SourceProductBaseCode=PW,SS
  Scope : Scope
  P : PMIOPort  Side=Left
  Pressure : Outport
  wires:
  PS-Simulink Converter/1 -> Gain/1
  Gain/1 -> Pressure/1, Scope/1  "Pressure"
  connections:
  PS-Simulink Converter/LConn1 -- Hydraulic Pressure Sensor/RConn2
  Hydraulic Reference2/LConn1 -- Hydraulic Pressure Sensor/RConn1
  Hydraulic Pressure Sensor/LConn1 -- P/RConn1

== system windEmulatorStep3/HPTOModel/HPTO/Subsystem ==
  Gain : Gain  Gain=60/(2*pi)
  Ideal Rotational Motion Sensor : fl_lib/Mechanical/Mechanical Sensors/Ideal Rotational Motion Sensor  wrap_angle=simscape.enum.onoff.off  offset=0 rad
  Mechanical Rotational Reference2 : fl_lib/Mechanical/Rotational Elements/Mechanical Rotational Reference
  PS Terminator : fl_lib/Physical Signals/Sinks/PS Terminator
  PS-Simulink Converter : nesl_utility/PS-Simulink Converter  PhysicalDomain=network_engine_domain  SubClassName=ps_output  LeftPortType=input  RightPortType=output  PseudoPeriodic=off  Frequencies=[]  Unit=inherit  AffineConversion=off
      settings: SourceProductBaseCode=PW,SS
  w : PMIOPort  Side=Left
  wShaft : Outport
  wires:
  PS-Simulink Converter/1 -> Gain/1
  Gain/1 -> wShaft/1  "ShaftSpeedMotor"
  connections:
  PS-Simulink Converter/LConn1 -- Ideal Rotational Motion Sensor/RConn2
  PS Terminator/LConn1 -- Ideal Rotational Motion Sensor/RConn3
  w/RConn1 -- Ideal Rotational Motion Sensor/LConn1
  Mechanical Rotational Reference2/LConn1 -- Ideal Rotational Motion Sensor/RConn1

== system windEmulatorStep3/HPTOModel/HPTO/Subsystem1 ==
  In1 : Inport
  Gain : Gain  Gain=0.0075
  LTI System2 : cstblocks/LTI System  sys=tf(100*2*pi,[1 200*pi])  IC=[]
  Out1 : Outport
  wires:
  LTI System2/1 -> Gain/1
  In1/1 -> LTI System2/1
  Gain/1 -> Out1/1

== system windEmulatorStep3/HPTOModel/HPTO/Subsystem2 ==
  1 : Inport
  Gain : Gain  Gain=0.0075
  LTI System2 : cstblocks/LTI System  sys=tf(100*2*pi,[1 200*pi])  IC=[]
  Out1 : Outport
  wires:
  LTI System2/1 -> Gain/1
  1/1 -> LTI System2/1
  Gain/1 -> Out1/1

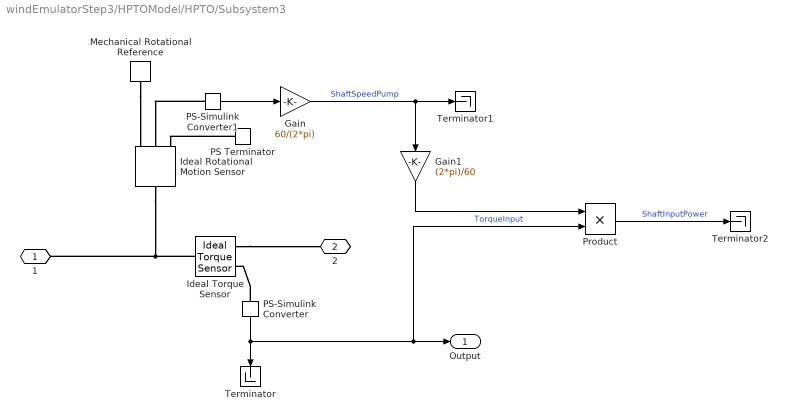
== system windEmulatorStep3/HPTOModel/HPTO/Subsystem3 ==
  Gain : Gain  Gain=60/(2*pi)
  Gain1 : Gain  Gain=(2*pi)/60
  Ideal Rotational Motion Sensor : fl_lib/Mechanical/Mechanical Sensors/Ideal Rotational Motion Sensor  wrap_angle=simscape.enum.onoff.off  offset=0 rad
  Ideal Torque Sensor : fl_lib/Mechanical/Mechanical Sensors/Ideal Torque Sensor
  Mechanical Rotational Reference : fl_lib/Mechanical/Rotational Elements/Mechanical Rotational Reference
  PS Terminator : fl_lib/Physical Signals/Sinks/PS Terminator
  PS-Simulink Converter : nesl_utility/PS-Simulink Converter  PhysicalDomain=network_engine_domain  SubClassName=ps_output  LeftPortType=input  RightPortType=output  PseudoPeriodic=off  Frequencies=[]  Unit=inherit  AffineConversion=off
      settings: SourceProductBaseCode=PW,SS
  PS-Simulink Converter1 : nesl_utility/PS-Simulink Converter  PhysicalDomain=network_engine_domain  SubClassName=ps_output  LeftPortType=input  RightPortType=output  PseudoPeriodic=off  Frequencies=[]  Unit=inherit  AffineConversion=off
      settings: SourceProductBaseCode=PW,SS
  Product : Product
  Terminator : Terminator
  Terminator1 : Terminator
  Terminator2 : Terminator
  1 : PMIOPort  Side=Left
  2 : PMIOPort  Port=2  Side=Right
  Output : Outport
  wires:
  PS-Simulink Converter/1 -> Terminator/1, Product/2, Output/1  "TorqueInput"
  Gain/1 -> Gain1/1, Terminator1/1  "ShaftSpeedPump"
  PS-Simulink Converter1/1 -> Gain/1
  Product/1 -> Terminator2/1  "ShaftInputPower"
  Gain1/1 -> Product/1
  connections:
  Ideal Rotational Motion Sensor/LConn1 -- Ideal Torque Sensor/LConn1 -- 1/RConn1
  Mechanical Rotational Reference/LConn1 -- Ideal Rotational Motion Sensor/RConn1
  PS Terminator/LConn1 -- Ideal Rotational Motion Sensor/RConn3
  PS-Simulink Converter1/LConn1 -- Ideal Rotational Motion Sensor/RConn2
  Ideal Torque Sensor/RConn1 -- 2/RConn1
  PS-Simulink Converter/LConn1 -- Ideal Torque Sensor/RConn2

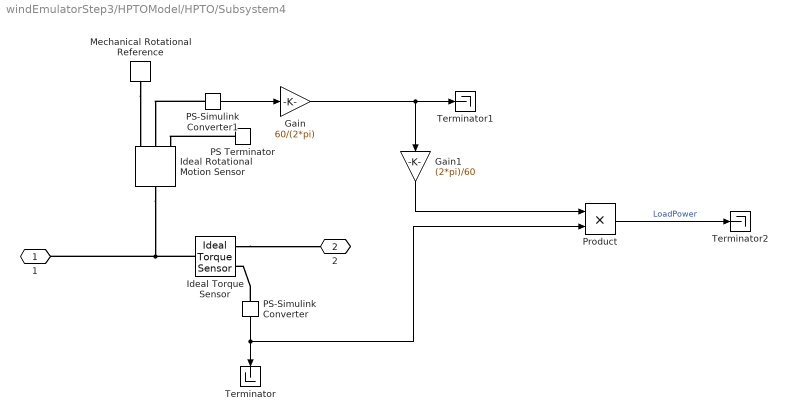
== system windEmulatorStep3/HPTOModel/HPTO/Subsystem4 ==
  Gain : Gain  Gain=60/(2*pi)
  Gain1 : Gain  Gain=(2*pi)/60
  Ideal Rotational Motion Sensor : fl_lib/Mechanical/Mechanical Sensors/Ideal Rotational Motion Sensor  wrap_angle=simscape.enum.onoff.off  offset=0 rad
  Ideal Torque Sensor : fl_lib/Mechanical/Mechanical Sensors/Ideal Torque Sensor
  Mechanical Rotational Reference : fl_lib/Mechanical/Rotational Elements/Mechanical Rotational Reference
  PS Terminator : fl_lib/Physical Signals/Sinks/PS Terminator
  PS-Simulink Converter : nesl_utility/PS-Simulink Converter  PhysicalDomain=network_engine_domain  SubClassName=ps_output  LeftPortType=input  RightPortType=output  PseudoPeriodic=off  Frequencies=[]  Unit=inherit  AffineConversion=off
      settings: SourceProductBaseCode=PW,SS
  PS-Simulink Converter1 : nesl_utility/PS-Simulink Converter  PhysicalDomain=network_engine_domain  SubClassName=ps_output  LeftPortType=input  RightPortType=output  PseudoPeriodic=off  Frequencies=[]  Unit=inherit  AffineConversion=off
      settings: SourceProductBaseCode=PW,SS
  Product : Product
  Terminator : Terminator
  Terminator1 : Terminator
  Terminator2 : Terminator
  1 : PMIOPort  Side=Left
  2 : PMIOPort  Port=2  Side=Right
  wires:
  PS-Simulink Converter/1 -> Terminator/1, Product/2
  Gain/1 -> Gain1/1, Terminator1/1
  PS-Simulink Converter1/1 -> Gain/1
  Product/1 -> Terminator2/1  "LoadPower"
  Gain1/1 -> Product/1
  connections:
  PS-Simulink Converter/LConn1 -- Ideal Torque Sensor/RConn2
  Ideal Torque Sensor/LConn1 -- Ideal Rotational Motion Sensor/LConn1 -- 1/RConn1
  Ideal Torque Sensor/RConn1 -- 2/RConn1
  Mechanical Rotational Reference/LConn1 -- Ideal Rotational Motion Sensor/RConn1
  PS Terminator/LConn1 -- Ideal Rotational Motion Sensor/RConn3
  PS-Simulink Converter1/LConn1 -- Ideal Rotational Motion Sensor/RConn2

== system windEmulatorStep3/HPTOModel/ControlAlgorithm/ForceToTorque/DesiredForce ==
  <LinearSpeedInput> : Inport
  <LinearPositionInput> : Inport  Port=2
  Add : Sum
  Constant : Constant  Value=Kdamping
  Constant1 : Constant  Value=Kpos
  Product : Product
  Product1 : Product
  ForceD : Outport
  wires:
  Add/1 -> ForceD/1  "ForceD"
  Constant1/1 -> Product1/2
  Constant/1 -> Product/1
  Product1/1 -> Add/2
  Product/1 -> Add/1
  <LinearPositionInput>/1 -> Product1/1
  <LinearSpeedInput>/1 -> Product/2

== system windEmulatorStep3/HPTOModel/ControlAlgorithm/PressureAbovePmin/PressureControl1 ==
  ActualPressure : Inport
  PressureRef : Inport  Port=2
  Add : Sum
  Discrete-Time Integrator : DiscreteIntegrator  SampleTime=-1  ICPrevOutput=DiscIntNeverNeededParam  ICPrevScaledInput=DiscIntNeverNeededParam
  Gain : Gain  Gain=PressureControl.PG
  Gain1 : Gain  Gain=PressureControl.IG
  Saturation : Saturate  UpperLimit=1  LowerLimit=-1
  Sum : Sum  Inputs=|-+
  ControlSignal2 : Outport
  wires:
  PressureRef/1 -> Sum/1
  ActualPressure/1 -> Sum/2
  Sum/1 -> Discrete-Time Integrator/1, Gain/1
  Gain/1 -> Add/1
  Discrete-Time Integrator/1 -> Gain1/1
  Gain1/1 -> Add/2
  Saturation/1 -> ControlSignal2/1
  Add/1 -> Saturation/1
